simulink model "P702_NI_SoftECU"  (R2019a)
settings: Solver=ode1  StartTime=0.0  StopTime=Inf  FixedStep=0.001  RelTol=1e-3  EnableMultiTasking=on
PreLoadFcn:
  | run '.\VeriStand_BlockSet\NIVeriStandAddPaths.m'
undefined symbols (not defined in the file or in its folder): magnitude
libraries: simulink x83, simulink_extras x1
(part 76 of 76)

== system P702_NI_SoftECU/SoftECU/SRR_L/RearLeft_SOD/SRR_RL_002/Subsystem/random_factor ==
  Range : Inport
  1-D Lookup Table : Lookup_n-D  NumberOfTableDimensions=1  BreakpointsForDimension1=[-10 10 20 40 80 1000]  Table="[1   1   1.2  2   3 3]"  InternalRulePriority=Speed  RndMeth=Simplest  InputSameDT=on
  Gain : Gain
  Product3 : Product  Inputs=3
  Random Number : RandomNumber  Variance=0.3  SampleTime=0.1
  Saturation : Saturate  UpperLimit=0.3  LowerLimit=-0.3
  Rand_Error : Outport
  wires:
  [Random_Status] -> Product3/3
  Saturation/1 -> Gain/1
  Product3/1 -> Rand_Error/1
  Range/1 -> 1-D Lookup Table/1
  1-D Lookup Table/1 -> Product3/1
  Gain/1 -> Product3/2
  Random Number/1 -> Saturation/1

== system P702_NI_SoftECU/SoftECU/SRR_L/RearLeft_SOD/SRR_RL_002/Subsystem/random_factor1 ==
  Range : Inport
  1-D Lookup Table : Lookup_n-D  NumberOfTableDimensions=1  BreakpointsForDimension1=[-10 10 20 40 80 1000]  Table="[1   1   1.2  2   3 3]"  InternalRulePriority=Speed  RndMeth=Simplest  InputSameDT=on
  Gain : Gain
  Product3 : Product  Inputs=3
  Random Number : RandomNumber  Variance=0.3  SampleTime=0.1
  Saturation : Saturate  UpperLimit=0.3  LowerLimit=-0.3
  Rand_Error : Outport
  wires:
  [Random_Status] -> Product3/3
  Saturation/1 -> Gain/1
  Product3/1 -> Rand_Error/1
  Range/1 -> 1-D Lookup Table/1
  1-D Lookup Table/1 -> Product3/1
  Gain/1 -> Product3/2
  Random Number/1 -> Saturation/1

== system P702_NI_SoftECU/SoftECU/SRR_L/RearLeft_SOD/SRR_RL_003/Subsystem/random_factor ==
  Range : Inport
  1-D Lookup Table : Lookup_n-D  NumberOfTableDimensions=1  BreakpointsForDimension1=[-10 10 20 40 80 1000]  Table="[1   1   1.2  2   3 3]"  InternalRulePriority=Speed  RndMeth=Simplest  InputSameDT=on
  Gain : Gain
  Product3 : Product  Inputs=3
  Random Number : RandomNumber  Variance=0.3  SampleTime=0.1
  Saturation : Saturate  UpperLimit=0.3  LowerLimit=-0.3
  Rand_Error : Outport
  wires:
  Random Number/1 -> Saturation/1
  Gain/1 -> Product3/2
  1-D Lookup Table/1 -> Product3/1
  Range/1 -> 1-D Lookup Table/1
  Product3/1 -> Rand_Error/1
  Saturation/1 -> Gain/1
  [Random_Status] -> Product3/3

== system P702_NI_SoftECU/SoftECU/SRR_L/RearLeft_SOD/SRR_RL_003/Subsystem/random_factor1 ==
  Range : Inport
  1-D Lookup Table : Lookup_n-D  NumberOfTableDimensions=1  BreakpointsForDimension1=[-10 10 20 40 80 1000]  Table="[1   1   1.2  2   3 3]"  InternalRulePriority=Speed  RndMeth=Simplest  InputSameDT=on
  Gain : Gain
  Product3 : Product  Inputs=3
  Random Number : RandomNumber  Variance=0.3  SampleTime=0.1
  Saturation : Saturate  UpperLimit=0.3  LowerLimit=-0.3
  Rand_Error : Outport
  wires:
  Random Number/1 -> Saturation/1
  Gain/1 -> Product3/2
  1-D Lookup Table/1 -> Product3/1
  Range/1 -> 1-D Lookup Table/1
  Product3/1 -> Rand_Error/1
  Saturation/1 -> Gain/1
  [Random_Status] -> Product3/3

== system P702_NI_SoftECU/SoftECU/SRR_R/FrontRight_SOD/SRR_FR_001 /Subsystem/random_factor ==
  Range : Inport
  1-D Lookup Table : Lookup_n-D  NumberOfTableDimensions=1  BreakpointsForDimension1=[-10 10 20 40 80 1000]  Table="[1   1   1.2  2   3 3]"  InternalRulePriority=Speed  RndMeth=Simplest  InputSameDT=on
  Gain : Gain
  Product3 : Product  Inputs=3
  Random Number : RandomNumber  Variance=0.3  SampleTime=0.1
  Saturation : Saturate  UpperLimit=0.3  LowerLimit=-0.3
  Rand_Error : Outport
  wires:
  [Random_Status] -> Product3/3
  Saturation/1 -> Gain/1
  Product3/1 -> Rand_Error/1
  Range/1 -> 1-D Lookup Table/1
  1-D Lookup Table/1 -> Product3/1
  Gain/1 -> Product3/2
  Random Number/1 -> Saturation/1

== system P702_NI_SoftECU/SoftECU/SRR_R/FrontRight_SOD/SRR_FR_001 /Subsystem/random_factor1 ==
  Range : Inport
  1-D Lookup Table : Lookup_n-D  NumberOfTableDimensions=1  BreakpointsForDimension1=[-10 10 20 40 80 1000]  Table="[1   1   1.2  2   3 3]"  InternalRulePriority=Speed  RndMeth=Simplest  InputSameDT=on
  Gain : Gain
  Product3 : Product  Inputs=3
  Random Number : RandomNumber  Variance=0.3  SampleTime=0.1
  Saturation : Saturate  UpperLimit=0.3  LowerLimit=-0.3
  Rand_Error : Outport
  wires:
  [Random_Status] -> Product3/3
  Saturation/1 -> Gain/1
  Product3/1 -> Rand_Error/1
  Range/1 -> 1-D Lookup Table/1
  1-D Lookup Table/1 -> Product3/1
  Gain/1 -> Product3/2
  Random Number/1 -> Saturation/1

== system P702_NI_SoftECU/SoftECU/SRR_R/FrontRight_SOD/SRR_FR_002/Subsystem/random_factor ==
  Range : Inport
  1-D Lookup Table : Lookup_n-D  NumberOfTableDimensions=1  BreakpointsForDimension1=[-10 10 20 40 80 1000]  Table="[1   1   1.2  2   3 3]"  InternalRulePriority=Speed  RndMeth=Simplest  InputSameDT=on
  Gain : Gain
  Product3 : Product  Inputs=3
  Random Number : RandomNumber  Variance=0.3  SampleTime=0.1
  Saturation : Saturate  UpperLimit=0.3  LowerLimit=-0.3
  Rand_Error : Outport
  wires:
  Random Number/1 -> Saturation/1
  Gain/1 -> Product3/2
  1-D Lookup Table/1 -> Product3/1
  Range/1 -> 1-D Lookup Table/1
  Product3/1 -> Rand_Error/1
  Saturation/1 -> Gain/1
  [Random_Status] -> Product3/3

== system P702_NI_SoftECU/SoftECU/SRR_R/FrontRight_SOD/SRR_FR_002/Subsystem/random_factor1 ==
  Range : Inport
  1-D Lookup Table : Lookup_n-D  NumberOfTableDimensions=1  BreakpointsForDimension1=[-10 10 20 40 80 1000]  Table="[1   1   1.2  2   3 3]"  InternalRulePriority=Speed  RndMeth=Simplest  InputSameDT=on
  Gain : Gain
  Product3 : Product  Inputs=3
  Random Number : RandomNumber  Variance=0.3  SampleTime=0.1
  Saturation : Saturate  UpperLimit=0.3  LowerLimit=-0.3
  Rand_Error : Outport
  wires:
  Random Number/1 -> Saturation/1
  Gain/1 -> Product3/2
  1-D Lookup Table/1 -> Product3/1
  Range/1 -> 1-D Lookup Table/1
  Product3/1 -> Rand_Error/1
  Saturation/1 -> Gain/1
  [Random_Status] -> Product3/3

== system P702_NI_SoftECU/SoftECU/SRR_R/FrontRight_SOD/SRR_FR_003/Subsystem/random_factor ==
  Range : Inport
  1-D Lookup Table : Lookup_n-D  NumberOfTableDimensions=1  BreakpointsForDimension1=[-10 10 20 40 80 1000]  Table="[1   1   1.2  2   3 3]"  InternalRulePriority=Speed  RndMeth=Simplest  InputSameDT=on
  Gain : Gain
  Product3 : Product  Inputs=3
  Random Number : RandomNumber  Variance=0.3  SampleTime=0.1
  Saturation : Saturate  UpperLimit=0.3  LowerLimit=-0.3
  Rand_Error : Outport
  wires:
  [Random_Status] -> Product3/3
  Saturation/1 -> Gain/1
  Product3/1 -> Rand_Error/1
  Range/1 -> 1-D Lookup Table/1
  1-D Lookup Table/1 -> Product3/1
  Gain/1 -> Product3/2
  Random Number/1 -> Saturation/1

== system P702_NI_SoftECU/SoftECU/SRR_R/FrontRight_SOD/SRR_FR_003/Subsystem/random_factor1 ==
  Range : Inport
  1-D Lookup Table : Lookup_n-D  NumberOfTableDimensions=1  BreakpointsForDimension1=[-10 10 20 40 80 1000]  Table="[1   1   1.2  2   3 3]"  InternalRulePriority=Speed  RndMeth=Simplest  InputSameDT=on
  Gain : Gain
  Product3 : Product  Inputs=3
  Random Number : RandomNumber  Variance=0.3  SampleTime=0.1
  Saturation : Saturate  UpperLimit=0.3  LowerLimit=-0.3
  Rand_Error : Outport
  wires:
  [Random_Status] -> Product3/3
  Saturation/1 -> Gain/1
  Product3/1 -> Rand_Error/1
  Range/1 -> 1-D Lookup Table/1
  1-D Lookup Table/1 -> Product3/1
  Gain/1 -> Product3/2
  Random Number/1 -> Saturation/1

== system P702_NI_SoftECU/SoftECU/SRR_R/RearRight_SOD/SRR_RR_001 /Subsystem/random_factor ==
  Range : Inport
  1-D Lookup Table : Lookup_n-D  NumberOfTableDimensions=1  BreakpointsForDimension1=[-10 10 20 40 80 1000]  Table="[1   1   1.2  2   3 3]"  InternalRulePriority=Speed  RndMeth=Simplest  InputSameDT=on
  Gain : Gain
  Product3 : Product  Inputs=3
  Random Number : RandomNumber  Variance=0.3  SampleTime=0.1
  Saturation : Saturate  UpperLimit=0.3  LowerLimit=-0.3
  Rand_Error : Outport
  wires:
  Random Number/1 -> Saturation/1
  Gain/1 -> Product3/2
  1-D Lookup Table/1 -> Product3/1
  Range/1 -> 1-D Lookup Table/1
  Product3/1 -> Rand_Error/1
  Saturation/1 -> Gain/1
  [Random_Status] -> Product3/3

== system P702_NI_SoftECU/SoftECU/SRR_R/RearRight_SOD/SRR_RR_001 /Subsystem/random_factor1 ==
  Range : Inport
  1-D Lookup Table : Lookup_n-D  NumberOfTableDimensions=1  BreakpointsForDimension1=[-10 10 20 40 80 1000]  Table="[1   1   1.2  2   3 3]"  InternalRulePriority=Speed  RndMeth=Simplest  InputSameDT=on
  Gain : Gain
  Product3 : Product  Inputs=3
  Random Number : RandomNumber  Variance=0.3  SampleTime=0.1
  Saturation : Saturate  UpperLimit=0.3  LowerLimit=-0.3
  Rand_Error : Outport
  wires:
  Random Number/1 -> Saturation/1
  Gain/1 -> Product3/2
  1-D Lookup Table/1 -> Product3/1
  Range/1 -> 1-D Lookup Table/1
  Product3/1 -> Rand_Error/1
  Saturation/1 -> Gain/1
  [Random_Status] -> Product3/3

== system P702_NI_SoftECU/SoftECU/SRR_R/RearRight_SOD/SRR_RR_002/Subsystem/random_factor ==
  Range : Inport
  1-D Lookup Table : Lookup_n-D  NumberOfTableDimensions=1  BreakpointsForDimension1=[-10 10 20 40 80 1000]  Table="[1   1   1.2  2   3 3]"  InternalRulePriority=Speed  RndMeth=Simplest  InputSameDT=on
  Gain : Gain
  Product3 : Product  Inputs=3
  Random Number : RandomNumber  Variance=0.3  SampleTime=0.1
  Saturation : Saturate  UpperLimit=0.3  LowerLimit=-0.3
  Rand_Error : Outport
  wires:
  [Random_Status] -> Product3/3
  Saturation/1 -> Gain/1
  Product3/1 -> Rand_Error/1
  Range/1 -> 1-D Lookup Table/1
  1-D Lookup Table/1 -> Product3/1
  Gain/1 -> Product3/2
  Random Number/1 -> Saturation/1

== system P702_NI_SoftECU/SoftECU/SRR_R/RearRight_SOD/SRR_RR_002/Subsystem/random_factor1 ==
  Range : Inport
  1-D Lookup Table : Lookup_n-D  NumberOfTableDimensions=1  BreakpointsForDimension1=[-10 10 20 40 80 1000]  Table="[1   1   1.2  2   3 3]"  InternalRulePriority=Speed  RndMeth=Simplest  InputSameDT=on
  Gain : Gain
  Product3 : Product  Inputs=3
  Random Number : RandomNumber  Variance=0.3  SampleTime=0.1
  Saturation : Saturate  UpperLimit=0.3  LowerLimit=-0.3
  Rand_Error : Outport
  wires:
  [Random_Status] -> Product3/3
  Saturation/1 -> Gain/1
  Product3/1 -> Rand_Error/1
  Range/1 -> 1-D Lookup Table/1
  1-D Lookup Table/1 -> Product3/1
  Gain/1 -> Product3/2
  Random Number/1 -> Saturation/1

== system P702_NI_SoftECU/SoftECU/SRR_R/RearRight_SOD/SRR_RR_003/Subsystem/random_factor ==
  Range : Inport
  1-D Lookup Table : Lookup_n-D  NumberOfTableDimensions=1  BreakpointsForDimension1=[-10 10 20 40 80 1000]  Table="[1   1   1.2  2   3 3]"  InternalRulePriority=Speed  RndMeth=Simplest  InputSameDT=on
  Gain : Gain
  Product3 : Product  Inputs=3
  Random Number : RandomNumber  Variance=0.3  SampleTime=0.1
  Saturation : Saturate  UpperLimit=0.3  LowerLimit=-0.3
  Rand_Error : Outport
  wires:
  Random Number/1 -> Saturation/1
  Gain/1 -> Product3/2
  1-D Lookup Table/1 -> Product3/1
  Range/1 -> 1-D Lookup Table/1
  Product3/1 -> Rand_Error/1
  Saturation/1 -> Gain/1
  [Random_Status] -> Product3/3

== system P702_NI_SoftECU/SoftECU/SRR_R/RearRight_SOD/SRR_RR_003/Subsystem/random_factor1 ==
  Range : Inport
  1-D Lookup Table : Lookup_n-D  NumberOfTableDimensions=1  BreakpointsForDimension1=[-10 10 20 40 80 1000]  Table="[1   1   1.2  2   3 3]"  InternalRulePriority=Speed  RndMeth=Simplest  InputSameDT=on
  Gain : Gain
  Product3 : Product  Inputs=3
  Random Number : RandomNumber  Variance=0.3  SampleTime=0.1
  Saturation : Saturate  UpperLimit=0.3  LowerLimit=-0.3
  Rand_Error : Outport
  wires:
  Random Number/1 -> Saturation/1
  Gain/1 -> Product3/2
  1-D Lookup Table/1 -> Product3/1
  Range/1 -> 1-D Lookup Table/1
  Product3/1 -> Rand_Error/1
  Saturation/1 -> Gain/1
  [Random_Status] -> Product3/3

== system P702_NI_SoftECU/SoftECU/PCM/Mapping/EngineData_7/FuelFlw_Vl_Dsply/Timer/Enabled Subsystem ==
  In1 : Inport
  Enable : EnablePort
  Out1 : Outport
  wires:
  In1/1 -> Out1/1

== system P702_NI_SoftECU/SoftECU/PCM/Mapping/EngineData_7/ODoCount/Timer/Enabled Subsystem ==
  In1 : Inport
  Enable : EnablePort
  Out1 : Outport
  wires:
  In1/1 -> Out1/1

== matlab function P702_NI_SoftECU/SoftECU/PCM/Logic1/Speed_Accel_Controller/MATLAB Function1 ==
  data: throttle_pos input; throttle output; cmbb_req input
function throttle = fcn(throttle_pos, cmbb_req)
if cmbb_req ~=0
    throttle = 0;
else
    throttle = throttle_pos;
end

== matlab function P702_NI_SoftECU/SoftECU/PCM/Logic1/Speed_Accel_Controller/MATLAB Function ==
  data: veh_speed input; desired_speed output; cmbb_req input; desired_speed_rq input; mrr input
function desired_speed = fcn(veh_speed, cmbb_req, desired_speed_rq, mrr)
if cmbb_req ~=0 || (veh_speed >= 5 && mrr<3 && mrr~=0)
    desired_speed = 0;
else
    desired_speed = desired_speed_rq;
end

== matlab function P702_NI_SoftECU/SoftECU/BCM/Logic/GGCC_Config_Mgmt_ID/VIN_Calculation ==
  data: Byte_0 output uint8; Byte_1 output uint8; Byte_2 output uint8; Byte_3 output uint8; Byte_4 output uint8; Byte_5 output uint8; Byte_6 output uint8; Byte_7 output uint8; VIN input; AxleRatio input; TireCircumference input; RCMAuxId input; MUX_out output; LowSpeedCmbbCfg input; FuelCfg input; AccCfg input; CmbbCfg input; DriveCfg input; DriveSideCfg input; GearboxCfg input; MUX_in input; C000_out output; C100_out output; C101_out output; C102_out output; C104_out output; C110_out output
function [Byte_0, Byte_1, Byte_2, Byte_3, Byte_4, Byte_5, Byte_6, Byte_7, MUX_out, C000_out, C100_out, C101_out, C102_out, C104_out, C110_out] = VIN_Calc(VIN, AxleRatio, TireCircumference, RCMAuxId, LowSpeedCmbbCfg, FuelCfg, AccCfg, CmbbCfg,  DriveCfg, DriveSideCfg, GearboxCfg, MUX_in)
% This block supports an embeddable subset of the MATLAB language.
% See the help menu for details. 

MUX_out = MUX_in + 1;

% Time
C000 = uint8([hex2dec('C0'), 0, 0, 0, 0, 0, 0, 0]);

% VIN
vinBytes = double(VIN);
C100 = uint8([hex2dec('C1') 0 vinBytes(1:6)]);
C101 = uint8([hex2dec('C1') 1 vinBytes(7:12)]);
C102 = uint8([hex2dec('C1') 2 vinBytes(13:17) 0]);

% Tire/Axle
% axleRatioBytes = flip(typecast(uint16(AxleRatio * 100), 'uint8'));
% tireCircBytes = flip(typecast(uint16(TireCircumference), 'uint8'));
% rcmAuxBytes = flip(typecast(uint16(RCMAuxId), 'uint8'));
axleRatioBytes = dec2bytepair(AxleRatio * 100);
tireCircBytes = dec2bytepair(TireCircumference);
rcmAuxBytes = dec2bytepair(RCMAuxId);
C104 = uint8([uint8(hex2dec('C1')) uint8(4) axleRatioBytes tireCircBytes rcmAuxBytes]);

% Config
cfg = bitshift(LowSpeedCmbbCfg, 46) + ...
    bitshift(FuelCfg, 39) + ...
    bitshift(AccCfg, 34) + ...
    bitshift(CmbbCfg, 29) + ...
    bitshift(DriveCfg, 21) + ...
    bitshift(DriveSideCfg, 18) + ...
    bitshift(GearboxCfg, 15);
cfg1 = bitshift(cfg, -32);
cfg2 = cfg-(cfg1 * 2^32);
cfgBytes = [flip(typecast(uint32(cfg1),'uint8')) flip(typecast(uint32(cfg2),'uint8'))];
cfgBytes = cfgBytes(3:8);
C110 = uint8([hex2dec('C1'), hex2dec('10'), cfgBytes]); 

% Test Out
C000_out = C000;
C100_out = C100;
C101_out = C101;
C102_out = C102;
C104_out = C104;
C110_out = C110;

switch MUX_in
    
    case 0 % Global vehicle time frame
        % TODO increment time
        Byte = C000;
        
    case 1 % VIN data frame 1
        Byte = C100;
        
    case 2 % VIN data frame 2
        Byte = C101;
        
    case 3 % VIN data frame 3
        Byte = C102;
        
    case 4 % Tire/Axle
        Byte = C104;
        
    case 5 % Config
        Byte = C110;
        MUX_out = 0;
    
    otherwise
        Byte = uint8([0, 0, 0, 0, 0, 0, 0, 0]);
                
end 
       
Byte_0 = Byte(1);
Byte_1 = Byte(2);
Byte_2 = Byte(3);
Byte_3 = Byte(4);
Byte_4 = Byte(5);
Byte_5 = Byte(6);
Byte_6 = Byte(7);
Byte_7 = Byte(8);

end

function bytepair = dec2bytepair(dec)
    byte1 = floor(dec / 2^8);
    byte2 = floor(dec - (byte1 * 2^8));
    bytepair = [byte1 byte2];
end

== matlab function P702_NI_SoftECU/SoftECU/RCM/Logic/Checksums/MATLAB Function ==
  data: VehRollYaw_No_Cnt input; RCM1_No_Cs output uint8; VehRol_W_Actl input; VehYaw_W_Actl input; VehRolWActl_Qf input; VehYawWActl_Qf input
function RCM1_No_Cs = Calc_VehRollYawW_No_Cs(VehRollYaw_No_Cnt, VehRol_W_Actl, VehYaw_W_Actl, VehRolWActl_Qf, VehYawWActl_Qf)
%Date Created: Apr 19 2011
%Author: John P. McCormick
%Purpose: Emulate RCM Checksum Calculator for Yaw & Roll Rate Signals
%% 4/20/2011, Added Long_Accel_Signal Input and revised the revised the Checksum Calculation
%% 4/20/2011, Added Long_Accel_Signal Input and revised the revised the Checksum Calculation
%% 4/21/2011, Revised the size of all the checksum parms to uint16. Why?
%%            Matlab limits the answer size of the sum(or any math operator) a bunch of Parmeters to the size of the smallest Parm(eg uint8 + uint16 = uint8). 
%%            Thus, even if the sum of the checksum parms was >255, Matlab clipped the answer to 255(0xFF). Thus, causing the Checksum = ~(0xFF) = 0x00.

% VehRol_W_Actl = 0; %Set to 0 rad/sec, since model does not emulate this signal
%VehRol_W_Actl_CAN = uint16((VehRol_W_Actl * 5000) + 32500);
VehRol_W_Actl_CAN = uint16((VehRol_W_Actl * 5000) + 32500);
VehRol_W_Actl_CAN_Hi_Byte = uint16(bitand(VehRol_W_Actl_CAN, 65280)/256);
VehRol_W_Actl_CAN_Lo_Byte = uint16(bitand(VehRol_W_Actl_CAN, 255));

% VehYaw_W_Actl = 0; %Set to 0 rad/sec, since model does not emulate this signal
VehYaw_W_Actl_CAN = uint16((VehYaw_W_Actl * 5000) + 32500);
VehYaw_W_Actl_CAN_Hi_Byte = uint16(bitand(VehYaw_W_Actl_CAN, 65280)/256);
VehYaw_W_Actl_CAN_Lo_Byte = uint16(bitand(VehYaw_W_Actl_CAN, 255));

VehRolWActl_D_Qf = uint16(VehRolWActl_Qf);
VehYawWActl_D_Qf = uint16(VehYawWActl_Qf);

Summed_Parms = VehRol_W_Actl_CAN_Hi_Byte + VehRol_W_Actl_CAN_Lo_Byte + VehYaw_W_Actl_CAN_Hi_Byte + ...
               VehYaw_W_Actl_CAN_Lo_Byte + VehRolWActl_D_Qf + VehYawWActl_D_Qf + uint16(VehRollYaw_No_Cnt);
RCM1_No_Cs = uint8(bitcmp(double(bitand(Summed_Parms, 255)), 'uint8'));

== matlab function P702_NI_SoftECU/SoftECU/RCM/Logic/Checksums/MATLAB Function1 ==
  data: VehLatLongVert_No_Cnt input; RCM2_No_Cs output uint8; VehLat2_A_Actl input; VehLong2_A_Actl input; VehVert2_A_Actl input; VehLatAActl_Qf input; VehLongAActl_Qf input; VehVertAActl_Qf input
function RCM2_No_Cs = Calc_VehLatLongVertA_No_Cs(VehLatLongVert_No_Cnt, VehLat2_A_Actl, VehLong2_A_Actl, VehVert2_A_Actl, VehLatAActl_Qf, VehLongAActl_Qf, VehVertAActl_Qf)
%Date Created: Apr 19 2011
%Author: John P. McCormick
%Purpose: Emulate RCM Checksum Calculator for Yaw & Roll Rate Signals
%% 4/20/2011, Added Long_Accel_Signal Input and revised the revised the Checksum Calculation
%% 4/20/2011, Added Long_Accel_Signal Input and revised the revised the Checksum Calculation
%% 4/21/2011, Revised the size of all the checksum parms to uint16. Why?
%%            Matlab limits the answer size of the sum(or any math operator) a bunch of Parmeters to the size of the smallest Parm(eg uint8 + uint16 = uint8). 
%%            Thus, even if the sum of the checksum parms was >255, Matlab clipped the answer to 255(0xFF). Thus, causing the Checksum = ~(0xFF) = 0x00.

% VehLat2_A_Actl = 0; %Set to 0 rad/sec, since model does not emulate this signal
VehLat2_A_Actl_CAN = uint16((VehLat2_A_Actl * 100) + 4000);
VehLat2_A_Actl_CAN_Hi_Byte = uint16(bitand(VehLat2_A_Actl_CAN, 65280)/256);
VehLat2_A_Actl_CAN_Lo_Byte = uint16(bitand(VehLat2_A_Actl_CAN, 255));

% VehLong2_A_Actl = 0; %Set to 0 rad/sec, since model does not emulate this signal
VehLong2_A_Actl_CAN = uint16((VehLong2_A_Actl * 100) + 4000);
VehLong2_A_Actl_CAN_Hi_Byte = uint16(bitand(VehLong2_A_Actl_CAN, 65280)/256);
VehLong2_A_Actl_CAN_Lo_Byte = uint16(bitand(VehLong2_A_Actl_CAN, 255));

% VehVert2_A_Actl = 0; %Set to 0 rad/sec, since model does not emulate this signal
VehVert2_A_Actl_CAN = uint16((VehVert2_A_Actl * 100) + 4000);
VehVert2_A_Actl_CAN_Hi_Byte = uint16(bitand(VehVert2_A_Actl_CAN, 65280)/256);
VehVert2_A_Actl_CAN_Lo_Byte = uint16(bitand(VehVert2_A_Actl_CAN, 255));

VehLatAActl_D_Qf = uint16(VehLatAActl_Qf);
VehLongAActl_D_Qf = uint16(VehLongAActl_Qf);
VehVertAActl_D_Qf = uint16(VehVertAActl_Qf);

Summed_Parms = VehLat2_A_Actl_CAN_Hi_Byte + VehLat2_A_Actl_CAN_Lo_Byte + VehLong2_A_Actl_CAN_Hi_Byte + ...
               VehLong2_A_Actl_CAN_Lo_Byte + VehVert2_A_Actl_CAN_Hi_Byte + VehVert2_A_Actl_CAN_Lo_Byte + VehLatAActl_D_Qf + VehLongAActl_D_Qf + VehVertAActl_D_Qf+ uint16(VehLatLongVert_No_Cnt);
RCM2_No_Cs = uint8(bitcmp(double(bitand(Summed_Parms, 255)), 'uint8'));

== matlab function P702_NI_SoftECU/SoftECU/PSCM/Logic/Checksums/MATLAB Function ==
  data: SteWhlRelInit2_An_Sns input; SteWhlOSRelInit2An_Est input; SteWhlAn_No_Cnt input; SteWhlRelCalib_An_Sns input; CD4_SteeringAngleCS output uint8; StePw_Rq input
function CD4_SteeringAngleCS = Calc_SteWhlAn_No_Cs(SteWhlRelInit2_An_Sns, SteWhlOSRelInit2An_Est , SteWhlAn_No_Cnt, SteWhlRelCalib_An_Sns, StePw_Rq)
%Date Created: Apr 13 2012
%Author: John P. McCormick
%Purpose: Emulate CD4 Program Steering Angle Checksum Calculator 

%Rev History
%% 4/12/2012, Started with the C1 Steering Wheel Checksum Calculator, but added a general CS Calculator
%% 2/8/2012, Added this new function from an Older RCM Checksum Calculator
%% 4/20/2011, Added Long_Accel_Signal Input and revised the revised the Checksum Calculation
%% 4/21/2011, Revised the size of all the checksum parms to uint16. Why?
%%            Matlab limits the answer size of the sum(or any math operator) a bunch of Parmeters to the size of the smallest Parm(eg uint8 + uint16 = uint8). 
%%            Thus, even if the sum of the checksum parms was >255, Matlab clipped the answer to 255(0xFF). Thus, causing the Checksum = ~(0xFF) = 0x00.

SteWhlRelInit2_An_Sns_Counts = uint16((SteWhlRelInit2_An_Sns * 10) + 32000); 
SteWhlOSRelInit2An_Est_Counts = uint16((SteWhlOSRelInit2An_Est * 10) + 32000); 
SteWhlRelInit2_An_Sns_MSB = uint16(bitand(SteWhlRelInit2_An_Sns_Counts, 65280)/256); 
SteWhlRelInit2_An_Sns_LSB = uint16(bitand(SteWhlRelInit2_An_Sns_Counts, 255));
SteWhlOSRelInit2An_Est_MSB = uint16(bitand(SteWhlOSRelInit2An_Est_Counts, 65280)/256);
SteWhlOSRelInit2An_Est_LSB = uint16(bitand(SteWhlOSRelInit2An_Est_Counts, 255));
SteWhlAn_No_Cnt_As_Byte = uint16(SteWhlAn_No_Cnt);
%SteWhlRelCalib_An_Sns_Counts = uint16((SteWhlRelCalib_An_Sns * 10) + 16000);

%StePw_B_Rq = uint16(StePw_Rq);

Summed_Parms = SteWhlRelInit2_An_Sns_MSB + SteWhlRelInit2_An_Sns_LSB + SteWhlOSRelInit2An_Est_MSB + ...
               SteWhlOSRelInit2An_Est_LSB + SteWhlAn_No_Cnt_As_Byte;
CD4_SteeringAngleCS = uint8(bitcmp(double(bitand(Summed_Parms, 255)), 'uint8'));

== stateflow chart P702_NI_SoftECU/SoftECU/PCM/Logic1/States/PowerPackStatus ==
  state Off
    entry: PowerPackStatus =100
    EngineState = 0
    Eng_D_Stat = 0
    PwPckTq_D_Stat = 0
    EngineSpeed = 0
    CrankingStatus=0
  state Init
    entry: PowerPackStatus = 101
    EngineState = 0
    Eng_D_Stat = 0
    PwPckTq_D_Stat = 0
  state Ready_2
    entry: PowerPackStatus = 103
    EngineState = 1
    Eng_D_Stat = 0
    PwPckTq_D_Stat = 0
    StartStopTimer = 0
  state Awake_1
    entry: PowerPackStatus = 102
    EngineState = 1
    Eng_D_Stat = 0
    PwPckTq_D_Stat = 0
  state PreStarting_3
    entry: PowerPackStatus = 104
    EngineState = 2
    Eng_D_Stat = 0
    PwPckTq_D_Stat = 2
  state StartInProgress_4
    entry: PowerPackStatus = 105
    EngineState = 2
    Eng_D_Stat = 0
    PwPckTq_D_Stat = 2
    CrankingStatus=1
    EngineSpeed = min(CrankDuration - TimeToStart,EngineSpeed_Running)
  state Running_Running_5_
    entry: PowerPackStatus = 106
    EngineState = 3
    Eng_D_Stat = 1
    PwPckTq_D_Stat = 3
    CrankingStatus=0
    EngineSpeed = EngineSpeed_Running
  state Running_Running_5
    entry: PowerPackStatus = 107
    EngineState = 3
    Eng_D_Stat = 1
    PwPckTq_D_Stat = 3
    EngineSpeed = EngineSpeed_Running
    CrankingStatus=0
    InProgTimer = 0
    InProgDelTimer = 0
  state Pre_Standby
  state StartStop_Timer
  state Running_Standby
    entry: PowerPackStatus = 6
    EngineSpeed = 0
  state Cranking_Status
    entry:CrankingStatus=1
  state StartingInProgress
    entry: PowerPackStatus = 7
    StartStopTimer = 0
    CrankingStatus=(InProgTimer<(CrankingStatusTimer-InProgDelTimer))
    EngineSpeed = min(InProgTimer/2,EngineSpeed_Running)
  state AfterRun_9
    entry: PowerPackStatus = 9
    EngineState = 5
    Eng_D_Stat = 0
    PwPckTq_D_Stat = 0
    EngineSpeed = 0
    InProgTimer = 0
    StartStopTimer = 0
    CrankingStatus=0
  state ShutOff
    entry: PowerPackStatus = 0
    EngineState = 6
    Eng_D_Stat = 0
    PwPckTq_D_Stat = 0
  (default) -> Off
  Init -> Init [order 3] : {PowerOnInitTimer -= 1}
  Off -> Init : [TE15 == 1 | EngineHW_Wakeup == 1]
      | {PowerOnInitTimer = 1000}
  Init -> Off [order 2] : [TE15 == 0 & EngineHW_Wakeup == 0]
  AfterRun_9 -> Init [order 2] : [TE15 == 1]
  Init -> Awake_1 [order 4] : [TE15 == 0 & EngineHW_Wakeup == 1]
  Init -> Ready_2 [order 1] : [PowerOnInitTimer == 0 & TE15 == 1]
  ShutOff -> Awake_1 : [TE15 == 1 | EngineHW_Wakeup == 1]
  Awake_1 -> Ready_2 [order 1] : [TE15 == 1]
  AfterRun_9 -> Awake_1 [order 1] : [(TE15 == 0) & ...
      | (EngineHW_Wakeup == 1) & ...
      | (AfterRunTaskTimer <= 0)]
  Awake_1 -> AfterRun_9 [order 2] : [TE15 == 0 & EngineHW_Wakeup == 0]
  Ready_2 -> PreStarting_3 : [((KeyPosition == 3 & ...
      |  KvModuleActivated == 0) |...
      |  (ClutchSwitch == 1 & ...
      |  StartButton == 1 & ...
      | KvModuleActivated == 1))]
      | {TimeToLeavePrestart = 500}
  PreStarting_3 -> Ready_2 [order 1] : [(KeyPosition < 3 & ...
      | KvModuleActivated == 0) |...
      | ((ClutchSwitch == 0 | ...
      | StartButton == 0) & ...
      | (KvModuleActivated == 1))]
  PreStarting_3 -> PreStarting_3 [order 3] : {TimeToLeavePrestart -= 1}
  PreStarting_3 -> StartInProgress_4 [order 2] : [TimeToLeavePrestart <= 0]
      | {TimeToStart = CrankDuration}
  StartInProgress_4 -> StartInProgress_4 [order 2] : {TimeToStart -= 1}
  StartInProgress_4 -> Running_Running_5_ [order 1] : [TimeToStart <= 0 & ...
      | KeyPosition <= 2]
  Running_Running_5_ -> Running_Running_5 : [ ((KvModuleActivated == 1) & (StartButton == 0))  | ...
      |   (KeyPosition <= 2 & KvModuleActivated == 0) ]
  Running_Running_5 -> Running_Running_5 [order 4] : {EngineSpeed = EngineSpeed_Running}
  Pre_Standby -> Running_Running_5 [order 2] : [(StartStop == 0) | (TE15 == 0)]
  Running_Running_5 -> StartStop_Timer [order 2] : [(StartStopTimer) < 5002 & (StartStop == 1)]
  Running_Running_5 -> Pre_Standby [order 3] : [(StartStop ==1)&(StartStopTimer > 5000)&(StSt_Inhibition==0)]
  StartStop_Timer -> Running_Running_5 : {StartStopTimer += 1}
  Pre_Standby -> Running_Standby [order 1] : [(StartStop == 1) & ...
      | (ClutchSwitch == 0) & ...
      | (VehicleSpeed<=2)]
  StartingInProgress -> Running_Running_5 [order 2] : [InProgTimer > StartingInProgressTimer]
  Running_Running_5 -> AfterRun_9 [order 1] : [TE15 == 0 | ...
      | (KvModuleActivated == 1 & ...
      | StartButton == 1)]
      | {AfterRunTaskTimer = 10000}
  StartingInProgress -> StartingInProgress [order 3] : {InProgTimer += 1}
  Running_Standby -> Cranking_Status [order 2] : [(ClutchSwitch == 1) | ...
      | (StSt_Inhibition==2)]
  Cranking_Status -> StartingInProgress [order 2] : [InProgDelTimer > StartingInProgressDelay]
  Cranking_Status -> Cranking_Status [order 3] : {InProgDelTimer += 1}
  Cranking_Status -> AfterRun_9 [order 1] : [TE15 == 0 | ...
      | (KvModuleActivated == 1 & ...
      | StartButton == 1)]
  Running_Standby -> AfterRun_9 [order 1] : [TE15 == 0 | ...
      | (KvModuleActivated == 1 & ...
      | StartButton == 1)]
  StartingInProgress -> AfterRun_9 [order 1] : [(TE15 == 0 & InProgTimer < 250) | ...
      | (KvModuleActivated == 1 & StartButton == 1)]
  AfterRun_9 -> AfterRun_9 [order 4] : {AfterRunTaskTimer-=1}
  AfterRun_9 -> ShutOff [order 3] : [AfterRunTaskTimer == 0 & TE15 == 0 & EngineHW_Wakeup == 0]
  data: EngineHW_Wakeup input boolean; ClutchSwitch input boolean; PowerPackStatus output uint8; KeyPosition input; TimeToLeavePrestart local double; TimeToStart local double; AfterRunTaskTimer local double; PowerOnInitTimer local double; TE15 input boolean; StartButton input boolean; KvModuleActivated input boolean; VehicleSpeed input; EngineSpeed_Running input double =1000; EngineState output double; StartStop input; CrankDuration input double; StartStopTimer local double; InProgTimer local double; StartingInProgressTimer input double [0..10000]; CrankingStatus output double; StartingInProgressDelay input double; CrankingStatusTimer input double; InProgDelTimer local double; EngineSpeed output double [0..8000]; StSt_Inhibition input double; Eng_D_Stat output double; PwPckTq_D_Stat output double

== stateflow chart P702_NI_SoftECU/SoftECU/ECM/Mapping/EngBrakeData/ReValueStates/Model_ACC_State ==
  state Wait/
  state Assign/
  state Enable/
  state Action/
    en: DeactivateSupply=1;
    FirstUse=0;
  state CheckDuration/
  state DontCare/
  (default) -> Enable : {DeactivateSupply=0;FirstUse=1;}
  Wait -> Assign [order 1] : [CurrState]
      | {DeactivateSupply=0;}
  Enable -> Wait [order 1] : [(EnableCurrCheck) && ((!CurrState)||(FirstUse))]
  Assign -> CheckDuration : after(CurrentCheckDuration,tick) % One tick = StepSize (1ms)
      | %Duration 500ms
  CheckDuration -> Action [order 1] : [CurrState]
  (junction 41) -> Wait
  Wait -> (junction 35) [order 2] : [Reset]
      | {DeactivateSupply=0;FirstUse=1;}
  (junction 37) -> Enable
  (junction 23) -> Enable
  Enable -> (junction 24) [order 2] : [(EnableCurrCheck)&&...
      | (CurrState)&&...
      | (!FirstUse)]
      | % !FirstUse: to avoid same
      | % transition conditions
  CheckDuration -> DontCare [order 2] : [!CurrState]
  (junction 25) -> Action
  Action -> (junction 22)
  DontCare -> (junction 41)
  (junction 24) -> (junction 25)
  (junction 22) -> (junction 23)
  (junction 35) -> (junction 37)
  data: a local double; DeactivateSupply output boolean; CurrState input; EnableCurrCheck input; FirstUse local double; CurrentCheckDuration input double; Reset input [0..1]

== stateflow chart P702_NI_SoftECU/SoftECU/ECM/Mapping/EngBrakeData/ReValueStates/AccStopModeRequest ==
  settings: updateMethod=DISCRETE  sampleTime=.001
  state Default
    en:
    AccStopMde_D_Rq=0;
    PrplTqMnSat_B_Actl_Reset =1;
  state wait_AccStopMde
  state setAccStopMde_D_Rq
    en:
    AccStopMde_D_Rq = 3;
    PrplTqMnSat_B_Actl_Reset =0;
  state wait_3_Sec
  (default) -> Default : {firsttime =1;}
  Default -> wait_AccStopMde [order 1] : [(AccStopStat_B_Rq && firsttime)]
  Default -> Default [order 2] : [reset]{firsttime=1;}
  wait_AccStopMde -> Default [order 1] : [reset]{firsttime = 1;}
  wait_AccStopMde -> wait_3_Sec [order 2] : [AccStopMde_Temp]
  setAccStopMde_D_Rq -> Default [order 1] : [AccResume]
      | {firsttime = 0;}
  setAccStopMde_D_Rq -> Default [order 2] : [reset]
      | {firsttime = 1;}
  wait_3_Sec -> setAccStopMde_D_Rq : after(StopModeDuration,tick)
      | % One {tick = StepSize} (1ms)
      | %Duration 500ms
  data: AccStopMde_D_Rq output double [0..5] =0; AccResume input boolean [0..1]; AccStopMde_Temp input boolean [0..1]; AccStopStat_B_Rq input boolean [0..1]; reset input boolean [0..1]; StopModeDuration input uint16 [0..3000]; firsttime local boolean [0..1]; PrplTqMnSat_B_Actl_Reset output boolean
  data AccStopMde_D_Rq settings: updateMethod=SF_CONTINUOUS_TIME_DATA
